simulink model "sm_stewart_platform"  (R2019b)
settings: Solver=ode45  StartTime=0.0  StopTime=450  MaxStep=0.2  RelTol=1e-3  EnableMultiTasking=on
model workspace (MAT data in the model file):
  g_density = 5
values from neighbouring files (symbols this model uses):
  B = base_points.Data(:,:,1)    [run_this_for_sim.m]
  base_radius = 0.75*100    (= 75)    [run_this_for_sim.m]
  desired_max_angle = 10    [run_this_for_sim.m]
  desired_max_x = 0.05    [run_this_for_sim.m]
  desired_max_y = desired_max_x    (= 0.05)    [run_this_for_sim.m]
  desired_max_z = 0.05    [run_this_for_sim.m]
  initial_integral_force = 200    [run_this_for_sim.m]
  leg_max = leg_min+0.3    (= 1.322)    [run_this_for_sim.m]
  leg_min = 1.022    [run_this_for_sim.m]
  leg_thickness = 75/1000    (= 0.075)    [run_this_for_sim.m]
  lower_leg_length = upper_leg_length    (= 0.511)    [run_this_for_sim.m]
  max_velocity = 0.15    [run_this_for_sim.m]
  P = platform_points.Data(:,:,1)    [run_this_for_sim.m]
  platform_radius = 0.75*base_radius    (= 56.25)    [run_this_for_sim.m]
  platform_thickness = 0.1/8    (= 0.0125)    [run_this_for_sim.m]
  trajectory_smoothing = 1/1.5    (= 0.666666666667)    [run_this_for_sim.m]
  upper_leg_length = dead_length/2    (= 0.511)    [run_this_for_sim.m]
  work_height = 1.2*100    (= 120)    [run_this_for_sim.m]
undefined symbols (not defined in the file or in its folder): nom_length, X, Z
libraries: sp_lib x18, nesl_utility x11, sm_lib x9, simulink x2
(part 10 of 10)

== system sm_stewart_platform/Subsystem/Reference Trajectory Generator7/Euler XYZ ==
  angles : Inport
  11 : Fcn  Expr=cos(u[2])*cos(u[3])
  12 : Fcn  Expr=-cos(u[2])*sin(u[3])
  13 : Fcn  Expr=sin(u[2])
  21 : Fcn  Expr=cos(u[3])*sin(u[2])*sin(u[1])+cos(u[1])*sin(u[3])
  22 : Fcn  Expr=cos(u[1])*cos(u[3]) - sin(u[1])*sin(u[2])*sin(u[3])
  23 : Fcn  Expr=-sin(u[1])*cos(u[2])
  31 : Fcn  Expr=sin(u[1])*sin(u[3]) - cos(u[1])*cos(u[3])*sin(u[2])
  32 : Fcn  Expr=cos(u[3])*sin(u[1])+cos(u[1])*sin(u[2])*sin(u[3])
  33 : Fcn  Expr=cos(u[1])*cos(u[2])
  Mux2 : Mux  Inputs=9
  Reshape 9x1->3x3 : Reshape  OutputDimensionality=Customize  OutputDimensions=[3,3]
  R : Outport  VectorParamsAs1DForOutWhenUnconnected=off
  wires:
  angles/1 -> 23/1, 33/1, 13/1, 32/1, 22/1, 12/1, 31/1, 21/1, 11/1
  33/1 -> Mux2/9
  23/1 -> Mux2/8
  13/1 -> Mux2/7
  32/1 -> Mux2/6
  22/1 -> Mux2/5
  12/1 -> Mux2/4
  31/1 -> Mux2/3
  21/1 -> Mux2/2
  11/1 -> Mux2/1
  Mux2/1 -> Reshape 9x1->3x3/1
  Reshape 9x1->3x3/1 -> R/1

== system sm_stewart_platform/Subsystem/Reference Trajectory Generator7/Euler XYZ Derivative ==
  R : Inport
  a : Inport  Port=2
  a' : Inport  Port=3
  b' : Inport  Port=4
  c' : Inport  Port=5
  Add : Sum
  Gain : Gain  Gain=-1
  Matrix Concatenate : Concatenate  NumInputs=3  Mode=Multidimensional array  ConcatenateDimension=2
  Mux5 : Mux  Inputs=3
  Prod{1..2,4..5} (4 alike) : Product  RndMeth=Zero
  Prod3 : Product  Multiplication=Matrix(*)  RndMeth=Zero
  R1 : Selector  NumberOfDimensions=2  InputPortWidth=3  IndexOptions=Select all,Index vector (dialog)  Indices=[1 3],1  OutputSizes=1,1
  R2 : Selector  NumberOfDimensions=2  InputPortWidth=3  IndexOptions=Select all,Index vector (dialog)  Indices=[1 3],2  OutputSizes=1,1
  Skew Op : Subsystem
  Vector Concatenate : Concatenate  NumInputs=3  Mode=Multidimensional array
  Zero Col : Constant  Value=[0 0 0]'
  sin cos : Trigonometry  Operator=sincos
  R' : Outport  VectorParamsAs1DForOutWhenUnconnected=off
  wires:
  a/1 -> sin cos/1
  sin cos/1 -> Prod1/2
  sin cos/2 -> Prod2/2
  b'/1 -> Prod2/1, Prod1/1
  a'/1 -> Mux5/1
  Prod2/1 -> Mux5/2
  Prod1/1 -> Mux5/3
  Mux5/1 -> Skew Op/1(v)
  Vector Concatenate/1 -> Prod4/2, Gain/1
  R2/1 -> Prod4/1
  Gain/1 -> Prod5/2
  Zero Col/1 -> Matrix Concatenate/3
  Prod5/1 -> Matrix Concatenate/2
  Prod4/1 -> Matrix Concatenate/1
  R1/1 -> Prod5/1
  Prod3/1 -> Add/1
  Matrix Concatenate/1 -> Add/2
  Add/1 -> R'/1
  R/1 -> R1/1, Prod3/2, R2/1
  Skew Op/1(v~) -> Prod3/1
  c'/1 -> Vector Concatenate/2, Vector Concatenate/1, Vector Concatenate/3

== system sm_stewart_platform/Subsystem/Reference Trajectory Generator7/Rx sinusoid ==
  t : Inport
  Add : Sum  Inputs=|++
  Add2 : Sum  Inputs=++|
  amp1 : Gain  Gain=A
  amp2 : Gain  Gain=w*A*pi/180
  deg2rad : Gain  Gain=pi/180
  freq : Gain  Gain=w
  offset : Constant  Value=k  VectorParams1D=off
  phase : Constant  Value=p  VectorParams1D=off
  sin cos : Trigonometry  Operator=sincos
  f : Outport  VectorParamsAs1DForOutWhenUnconnected=off
  f' : Outport  Port=2  VectorParamsAs1DForOutWhenUnconnected=off
  wires:
  t/1 -> freq/1
  Add/1 -> deg2rad/1
  phase/1 -> Add/2
  amp2/1 -> f'/1
  Add2/1 -> f/1
  offset/1 -> Add2/1
  sin cos/1 -> amp1/1
  sin cos/2 -> amp2/1
  amp1/1 -> Add2/2
  freq/1 -> Add/1
  deg2rad/1 -> sin cos/1

== system sm_stewart_platform/Subsystem/Reference Trajectory Generator7/Ry sinusoid ==
  t : Inport
  Add : Sum  Inputs=|++
  Add2 : Sum  Inputs=++|
  amp1 : Gain  Gain=A
  amp2 : Gain  Gain=w*A*pi/180
  deg2rad : Gain  Gain=pi/180
  freq : Gain  Gain=w
  offset : Constant  Value=k  VectorParams1D=off
  phase : Constant  Value=p  VectorParams1D=off
  sin cos : Trigonometry  Operator=sincos
  f : Outport  VectorParamsAs1DForOutWhenUnconnected=off
  f' : Outport  Port=2  VectorParamsAs1DForOutWhenUnconnected=off
  wires:
  t/1 -> freq/1
  Add/1 -> deg2rad/1
  phase/1 -> Add/2
  amp2/1 -> f'/1
  Add2/1 -> f/1
  offset/1 -> Add2/1
  sin cos/1 -> amp1/1
  sin cos/2 -> amp2/1
  amp1/1 -> Add2/2
  freq/1 -> Add/1
  deg2rad/1 -> sin cos/1

== system sm_stewart_platform/Subsystem/Reference Trajectory Generator7/Rz sinusoid ==
  t : Inport
  Add : Sum  Inputs=|++
  Add2 : Sum  Inputs=++|
  amp1 : Gain  Gain=A
  amp2 : Gain  Gain=w*A*pi/180
  deg2rad : Gain  Gain=pi/180
  freq : Gain  Gain=w
  offset : Constant  Value=k  VectorParams1D=off
  phase : Constant  Value=p  VectorParams1D=off
  sin cos : Trigonometry  Operator=sincos
  f : Outport  VectorParamsAs1DForOutWhenUnconnected=off
  f' : Outport  Port=2  VectorParamsAs1DForOutWhenUnconnected=off
  wires:
  t/1 -> freq/1
  Add/1 -> deg2rad/1
  phase/1 -> Add/2
  amp2/1 -> f'/1
  Add2/1 -> f/1
  offset/1 -> Add2/1
  sin cos/1 -> amp1/1
  sin cos/2 -> amp2/1
  amp1/1 -> Add2/2
  freq/1 -> Add/1
  deg2rad/1 -> sin cos/1

== system sm_stewart_platform/Subsystem/Reference Trajectory Generator7/dx sinusoid ==
  t : Inport
  Add : Sum  Inputs=|++
  Add2 : Sum  Inputs=++|
  amp1 : Gain  Gain=A
  amp2 : Gain  Gain=w*A*pi/180
  deg2rad : Gain  Gain=pi/180
  freq : Gain  Gain=w
  offset : Constant  Value=k  VectorParams1D=off
  phase : Constant  Value=p  VectorParams1D=off
  sin cos : Trigonometry  Operator=sincos
  f : Outport  VectorParamsAs1DForOutWhenUnconnected=off
  f' : Outport  Port=2  VectorParamsAs1DForOutWhenUnconnected=off
  wires:
  t/1 -> freq/1
  Add/1 -> deg2rad/1
  phase/1 -> Add/2
  amp2/1 -> f'/1
  Add2/1 -> f/1
  offset/1 -> Add2/1
  sin cos/1 -> amp1/1
  sin cos/2 -> amp2/1
  amp1/1 -> Add2/2
  freq/1 -> Add/1
  deg2rad/1 -> sin cos/1

== system sm_stewart_platform/Subsystem/Reference Trajectory Generator7/dy sinusoid ==
  t : Inport
  Add : Sum  Inputs=|++
  Add2 : Sum  Inputs=++|
  amp1 : Gain  Gain=A
  amp2 : Gain  Gain=w*A*pi/180
  deg2rad : Gain  Gain=pi/180
  freq : Gain  Gain=w
  offset : Constant  Value=k  VectorParams1D=off
  phase : Constant  Value=p  VectorParams1D=off
  sin cos : Trigonometry  Operator=sincos
  f : Outport  VectorParamsAs1DForOutWhenUnconnected=off
  f' : Outport  Port=2  VectorParamsAs1DForOutWhenUnconnected=off
  wires:
  t/1 -> freq/1
  Add/1 -> deg2rad/1
  phase/1 -> Add/2
  amp2/1 -> f'/1
  Add2/1 -> f/1
  offset/1 -> Add2/1
  sin cos/1 -> amp1/1
  sin cos/2 -> amp2/1
  amp1/1 -> Add2/2
  freq/1 -> Add/1
  deg2rad/1 -> sin cos/1

== system sm_stewart_platform/Subsystem/Reference Trajectory Generator7/dz sinusoid ==
  t : Inport
  Add : Sum  Inputs=|++
  Add2 : Sum  Inputs=++|
  amp1 : Gain  Gain=A
  amp2 : Gain  Gain=w*A*pi/180
  deg2rad : Gain  Gain=pi/180
  freq : Gain  Gain=w
  offset : Constant  Value=k  VectorParams1D=off
  phase : Constant  Value=p  VectorParams1D=off
  sin cos : Trigonometry  Operator=sincos
  f : Outport  VectorParamsAs1DForOutWhenUnconnected=off
  f' : Outport  Port=2  VectorParamsAs1DForOutWhenUnconnected=off
  wires:
  t/1 -> freq/1
  Add/1 -> deg2rad/1
  phase/1 -> Add/2
  amp2/1 -> f'/1
  Add2/1 -> f/1
  offset/1 -> Add2/1
  sin cos/1 -> amp1/1
  sin cos/2 -> amp2/1
  amp1/1 -> Add2/2
  freq/1 -> Add/1
  deg2rad/1 -> sin cos/1

== system sm_stewart_platform/Subsystem/Reference Trajectory Generator8/Euler XYZ ==
  angles : Inport
  11 : Fcn  Expr=cos(u[2])*cos(u[3])
  12 : Fcn  Expr=-cos(u[2])*sin(u[3])
  13 : Fcn  Expr=sin(u[2])
  21 : Fcn  Expr=cos(u[3])*sin(u[2])*sin(u[1])+cos(u[1])*sin(u[3])
  22 : Fcn  Expr=cos(u[1])*cos(u[3]) - sin(u[1])*sin(u[2])*sin(u[3])
  23 : Fcn  Expr=-sin(u[1])*cos(u[2])
  31 : Fcn  Expr=sin(u[1])*sin(u[3]) - cos(u[1])*cos(u[3])*sin(u[2])
  32 : Fcn  Expr=cos(u[3])*sin(u[1])+cos(u[1])*sin(u[2])*sin(u[3])
  33 : Fcn  Expr=cos(u[1])*cos(u[2])
  Mux2 : Mux  Inputs=9
  Reshape 9x1->3x3 : Reshape  OutputDimensionality=Customize  OutputDimensions=[3,3]
  R : Outport  VectorParamsAs1DForOutWhenUnconnected=off
  wires:
  angles/1 -> 23/1, 33/1, 13/1, 32/1, 22/1, 12/1, 31/1, 21/1, 11/1
  33/1 -> Mux2/9
  23/1 -> Mux2/8
  13/1 -> Mux2/7
  32/1 -> Mux2/6
  22/1 -> Mux2/5
  12/1 -> Mux2/4
  31/1 -> Mux2/3
  21/1 -> Mux2/2
  11/1 -> Mux2/1
  Mux2/1 -> Reshape 9x1->3x3/1
  Reshape 9x1->3x3/1 -> R/1

== system sm_stewart_platform/Subsystem/Reference Trajectory Generator8/Euler XYZ Derivative ==
  R : Inport
  a : Inport  Port=2
  a' : Inport  Port=3
  b' : Inport  Port=4
  c' : Inport  Port=5
  Add : Sum
  Gain : Gain  Gain=-1
  Matrix Concatenate : Concatenate  NumInputs=3  Mode=Multidimensional array  ConcatenateDimension=2
  Mux5 : Mux  Inputs=3
  Prod{1..2,4..5} (4 alike) : Product  RndMeth=Zero
  Prod3 : Product  Multiplication=Matrix(*)  RndMeth=Zero
  R1 : Selector  NumberOfDimensions=2  InputPortWidth=3  IndexOptions=Select all,Index vector (dialog)  Indices=[1 3],1  OutputSizes=1,1
  R2 : Selector  NumberOfDimensions=2  InputPortWidth=3  IndexOptions=Select all,Index vector (dialog)  Indices=[1 3],2  OutputSizes=1,1
  Skew Op : Subsystem
  Vector Concatenate : Concatenate  NumInputs=3  Mode=Multidimensional array
  Zero Col : Constant  Value=[0 0 0]'
  sin cos : Trigonometry  Operator=sincos
  R' : Outport  VectorParamsAs1DForOutWhenUnconnected=off
  wires:
  a/1 -> sin cos/1
  sin cos/1 -> Prod1/2
  sin cos/2 -> Prod2/2
  b'/1 -> Prod2/1, Prod1/1
  a'/1 -> Mux5/1
  Prod2/1 -> Mux5/2
  Prod1/1 -> Mux5/3
  Mux5/1 -> Skew Op/1(v)
  Vector Concatenate/1 -> Prod4/2, Gain/1
  R2/1 -> Prod4/1
  Gain/1 -> Prod5/2
  Zero Col/1 -> Matrix Concatenate/3
  Prod5/1 -> Matrix Concatenate/2
  Prod4/1 -> Matrix Concatenate/1
  R1/1 -> Prod5/1
  Prod3/1 -> Add/1
  Matrix Concatenate/1 -> Add/2
  Add/1 -> R'/1
  R/1 -> R1/1, Prod3/2, R2/1
  Skew Op/1(v~) -> Prod3/1
  c'/1 -> Vector Concatenate/2, Vector Concatenate/1, Vector Concatenate/3

== system sm_stewart_platform/Subsystem/Reference Trajectory Generator8/Rx sinusoid ==
  t : Inport
  Add : Sum  Inputs=|++
  Add2 : Sum  Inputs=++|
  amp1 : Gain  Gain=A
  amp2 : Gain  Gain=w*A*pi/180
  deg2rad : Gain  Gain=pi/180
  freq : Gain  Gain=w
  offset : Constant  Value=k  VectorParams1D=off
  phase : Constant  Value=p  VectorParams1D=off
  sin cos : Trigonometry  Operator=sincos
  f : Outport  VectorParamsAs1DForOutWhenUnconnected=off
  f' : Outport  Port=2  VectorParamsAs1DForOutWhenUnconnected=off
  wires:
  t/1 -> freq/1
  Add/1 -> deg2rad/1
  phase/1 -> Add/2
  amp2/1 -> f'/1
  Add2/1 -> f/1
  offset/1 -> Add2/1
  sin cos/1 -> amp1/1
  sin cos/2 -> amp2/1
  amp1/1 -> Add2/2
  freq/1 -> Add/1
  deg2rad/1 -> sin cos/1

== system sm_stewart_platform/Subsystem/Reference Trajectory Generator8/Ry sinusoid ==
  t : Inport
  Add : Sum  Inputs=|++
  Add2 : Sum  Inputs=++|
  amp1 : Gain  Gain=A
  amp2 : Gain  Gain=w*A*pi/180
  deg2rad : Gain  Gain=pi/180
  freq : Gain  Gain=w
  offset : Constant  Value=k  VectorParams1D=off
  phase : Constant  Value=p  VectorParams1D=off
  sin cos : Trigonometry  Operator=sincos
  f : Outport  VectorParamsAs1DForOutWhenUnconnected=off
  f' : Outport  Port=2  VectorParamsAs1DForOutWhenUnconnected=off
  wires:
  t/1 -> freq/1
  Add/1 -> deg2rad/1
  phase/1 -> Add/2
  amp2/1 -> f'/1
  Add2/1 -> f/1
  offset/1 -> Add2/1
  sin cos/1 -> amp1/1
  sin cos/2 -> amp2/1
  amp1/1 -> Add2/2
  freq/1 -> Add/1
  deg2rad/1 -> sin cos/1

== system sm_stewart_platform/Subsystem/Reference Trajectory Generator8/Rz sinusoid ==
  t : Inport
  Add : Sum  Inputs=|++
  Add2 : Sum  Inputs=++|
  amp1 : Gain  Gain=A
  amp2 : Gain  Gain=w*A*pi/180
  deg2rad : Gain  Gain=pi/180
  freq : Gain  Gain=w
  offset : Constant  Value=k  VectorParams1D=off
  phase : Constant  Value=p  VectorParams1D=off
  sin cos : Trigonometry  Operator=sincos
  f : Outport  VectorParamsAs1DForOutWhenUnconnected=off
  f' : Outport  Port=2  VectorParamsAs1DForOutWhenUnconnected=off
  wires:
  t/1 -> freq/1
  Add/1 -> deg2rad/1
  phase/1 -> Add/2
  amp2/1 -> f'/1
  Add2/1 -> f/1
  offset/1 -> Add2/1
  sin cos/1 -> amp1/1
  sin cos/2 -> amp2/1
  amp1/1 -> Add2/2
  freq/1 -> Add/1
  deg2rad/1 -> sin cos/1

== system sm_stewart_platform/Subsystem/Reference Trajectory Generator8/dx sinusoid ==
  t : Inport
  Add : Sum  Inputs=|++
  Add2 : Sum  Inputs=++|
  amp1 : Gain  Gain=A
  amp2 : Gain  Gain=w*A*pi/180
  deg2rad : Gain  Gain=pi/180
  freq : Gain  Gain=w
  offset : Constant  Value=k  VectorParams1D=off
  phase : Constant  Value=p  VectorParams1D=off
  sin cos : Trigonometry  Operator=sincos
  f : Outport  VectorParamsAs1DForOutWhenUnconnected=off
  f' : Outport  Port=2  VectorParamsAs1DForOutWhenUnconnected=off
  wires:
  t/1 -> freq/1
  Add/1 -> deg2rad/1
  phase/1 -> Add/2
  amp2/1 -> f'/1
  Add2/1 -> f/1
  offset/1 -> Add2/1
  sin cos/1 -> amp1/1
  sin cos/2 -> amp2/1
  amp1/1 -> Add2/2
  freq/1 -> Add/1
  deg2rad/1 -> sin cos/1

== system sm_stewart_platform/Subsystem/Reference Trajectory Generator8/dy sinusoid ==
  t : Inport
  Add : Sum  Inputs=|++
  Add2 : Sum  Inputs=++|
  amp1 : Gain  Gain=A
  amp2 : Gain  Gain=w*A*pi/180
  deg2rad : Gain  Gain=pi/180
  freq : Gain  Gain=w
  offset : Constant  Value=k  VectorParams1D=off
  phase : Constant  Value=p  VectorParams1D=off
  sin cos : Trigonometry  Operator=sincos
  f : Outport  VectorParamsAs1DForOutWhenUnconnected=off
  f' : Outport  Port=2  VectorParamsAs1DForOutWhenUnconnected=off
  wires:
  t/1 -> freq/1
  Add/1 -> deg2rad/1
  phase/1 -> Add/2
  amp2/1 -> f'/1
  Add2/1 -> f/1
  offset/1 -> Add2/1
  sin cos/1 -> amp1/1
  sin cos/2 -> amp2/1
  amp1/1 -> Add2/2
  freq/1 -> Add/1
  deg2rad/1 -> sin cos/1

== system sm_stewart_platform/Subsystem/Reference Trajectory Generator8/dz sinusoid ==
  t : Inport
  Add : Sum  Inputs=|++
  Add2 : Sum  Inputs=++|
  amp1 : Gain  Gain=A
  amp2 : Gain  Gain=w*A*pi/180
  deg2rad : Gain  Gain=pi/180
  freq : Gain  Gain=w
  offset : Constant  Value=k  VectorParams1D=off
  phase : Constant  Value=p  VectorParams1D=off
  sin cos : Trigonometry  Operator=sincos
  f : Outport  VectorParamsAs1DForOutWhenUnconnected=off
  f' : Outport  Port=2  VectorParamsAs1DForOutWhenUnconnected=off
  wires:
  t/1 -> freq/1
  Add/1 -> deg2rad/1
  phase/1 -> Add/2
  amp2/1 -> f'/1
  Add2/1 -> f/1
  offset/1 -> Add2/1
  sin cos/1 -> amp1/1
  sin cos/2 -> amp2/1
  amp1/1 -> Add2/2
  freq/1 -> Add/1
  deg2rad/1 -> sin cos/1

== system sm_stewart_platform/Stewart Platform System/Inverse Kinematics Module/Pos Computation/6-Way Column Splitter ==
  A : Inport
  Column 1 : Selector  NumberOfDimensions=2  InputPortWidth=3  IndexOptions=Select all,Index vector (dialog)  Indices=-1,1  OutputSizes=1
  Column 2 : Selector  NumberOfDimensions=2  InputPortWidth=3  IndexOptions=Select all,Index vector (dialog)  Indices=-1,2  OutputSizes=1
  Column 3 : Selector  NumberOfDimensions=2  InputPortWidth=3  IndexOptions=Select all,Index vector (dialog)  Indices=-1,3  OutputSizes=1
  Column 4 : Selector  NumberOfDimensions=2  InputPortWidth=3  IndexOptions=Select all,Index vector (dialog)  Indices=-1,4  OutputSizes=1
  Column 5 : Selector  NumberOfDimensions=2  InputPortWidth=3  IndexOptions=Select all,Index vector (dialog)  Indices=-1,5  OutputSizes=1
  Column 6 : Selector  NumberOfDimensions=2  InputPortWidth=3  IndexOptions=Select all,Index vector (dialog)  Indices=-1,6  OutputSizes=1
  Col1 : Outport  VectorParamsAs1DForOutWhenUnconnected=off
  Col2 : Outport  Port=2  VectorParamsAs1DForOutWhenUnconnected=off
  Col3 : Outport  Port=3  VectorParamsAs1DForOutWhenUnconnected=off
  Col4 : Outport  Port=4  VectorParamsAs1DForOutWhenUnconnected=off
  Col5 : Outport  Port=5  VectorParamsAs1DForOutWhenUnconnected=off
  Col6 : Outport  Port=6  VectorParamsAs1DForOutWhenUnconnected=off
  wires:
  A/1 -> Column 3/1, Column 2/1, Column 1/1, Column 4/1, Column 5/1, Column 6/1
  Column 1/1 -> Col1/1
  Column 2/1 -> Col2/1
  Column 3/1 -> Col3/1
  Column 4/1 -> Col4/1
  Column 5/1 -> Col5/1
  Column 6/1 -> Col6/1

== system sm_stewart_platform/Stewart Platform System/Inverse Kinematics Module/Vel Computation/6-Way Column Splitter ==
  A : Inport
  Column 1 : Selector  NumberOfDimensions=2  InputPortWidth=3  IndexOptions=Select all,Index vector (dialog)  Indices=-1,1  OutputSizes=1
  Column 2 : Selector  NumberOfDimensions=2  InputPortWidth=3  IndexOptions=Select all,Index vector (dialog)  Indices=-1,2  OutputSizes=1
  Column 3 : Selector  NumberOfDimensions=2  InputPortWidth=3  IndexOptions=Select all,Index vector (dialog)  Indices=-1,3  OutputSizes=1
  Column 4 : Selector  NumberOfDimensions=2  InputPortWidth=3  IndexOptions=Select all,Index vector (dialog)  Indices=-1,4  OutputSizes=1
  Column 5 : Selector  NumberOfDimensions=2  InputPortWidth=3  IndexOptions=Select all,Index vector (dialog)  Indices=-1,5  OutputSizes=1
  Column 6 : Selector  NumberOfDimensions=2  InputPortWidth=3  IndexOptions=Select all,Index vector (dialog)  Indices=-1,6  OutputSizes=1
  Col1 : Outport  VectorParamsAs1DForOutWhenUnconnected=off
  Col2 : Outport  Port=2  VectorParamsAs1DForOutWhenUnconnected=off
  Col3 : Outport  Port=3  VectorParamsAs1DForOutWhenUnconnected=off
  Col4 : Outport  Port=4  VectorParamsAs1DForOutWhenUnconnected=off
  Col5 : Outport  Port=5  VectorParamsAs1DForOutWhenUnconnected=off
  Col6 : Outport  Port=6  VectorParamsAs1DForOutWhenUnconnected=off
  wires:
  A/1 -> Column 3/1, Column 2/1, Column 1/1, Column 4/1, Column 5/1, Column 6/1
  Column 1/1 -> Col1/1
  Column 2/1 -> Col2/1
  Column 3/1 -> Col3/1
  Column 4/1 -> Col4/1
  Column 5/1 -> Col5/1
  Column 6/1 -> Col6/1

== system sm_stewart_platform/Stewart Platform System/Manipulator/Base/Skewed Hexagon ==
  Solid : sm_lib/Body Elements/Extruded Solid  GraphicAmbientColor=0.1 * [1 1 1]  BasedOnType=Density  CenterOfMass=[0 0 0]  CenterOfMassUnits=m  GraphicDiffuseColor=diffuse  ExtrusionCrossSection=cross_sect  ExtrusionCrossSectionUnits=cm  Density=g_density  DensityUnits=g/cm^3  DoExposeReferenceFrame=on  GraphicEmissiveColor=[0 0 0]  ExportEntireGeometry=off  ExtrusionLength=thick  ExtrusionLengthUnits=cm  ExtrusionType=General  SerializedFrames=<Frames/>  MarkerShape=Sphere  MarkerSize=1  GraphicType=FromGeometry  InertiaType=CalculateFromGeometry  Mass=1  MassUnits=kg  MomentsOfInertia=[1 1 1]  MomentsOfInertiaUnits=kg*m^2  PolygonNumSides=1  GraphicOpacity=1  PolygonOuterRadius=1  PolygonOuterRadiusUnits=m  ProductsOfInertia=[0 0 0]  ProductsOfInertiaUnits=kg*m^2  GraphicShininess=shininess  GraphicSpecularColor=specular  GraphicVisPropType=AdvancedVisualProperties
      settings: SourceProductName=Simscape Multibody
  Conn1 : PMIOPort  Side=Right
  connections:
  Conn1/RConn1 -- Solid/RConn1

== system sm_stewart_platform/Stewart Platform System/Manipulator/Platform/Skewed Hexagon ==
  Solid : sm_lib/Body Elements/Extruded Solid  GraphicAmbientColor=0.1 * [1 1 1]  BasedOnType=Density  CenterOfMass=[0 0 0]  CenterOfMassUnits=m  GraphicDiffuseColor=diffuse  ExtrusionCrossSection=cross_sect  ExtrusionCrossSectionUnits=cm  Density=g_density  DensityUnits=g/cm^3  DoExposeReferenceFrame=on  GraphicEmissiveColor=[0 0 0]  ExportEntireGeometry=off  ExtrusionLength=thick  ExtrusionLengthUnits=cm  ExtrusionType=General  SerializedFrames=<Frames/>  MarkerShape=Sphere  MarkerSize=1  GraphicType=FromGeometry  InertiaType=CalculateFromGeometry  Mass=1  MassUnits=kg  MomentsOfInertia=[1 1 1]  MomentsOfInertiaUnits=kg*m^2  PolygonNumSides=1  GraphicOpacity=1  PolygonOuterRadius=1  PolygonOuterRadiusUnits=m  ProductsOfInertia=[0 0 0]  ProductsOfInertiaUnits=kg*m^2  GraphicShininess=shininess  GraphicSpecularColor=specular  GraphicVisPropType=AdvancedVisualProperties
      settings: SourceProductName=Simscape Multibody
  Conn1 : PMIOPort  Side=Right
  connections:
  Conn1/RConn1 -- Solid/RConn1

== system sm_stewart_platform/Subsystem/Reference Trajectory Generator/Euler XYZ Derivative/Skew Op ==
  v : Inport
  Demux : Demux  Outputs=3
  Demux1 : Demux  Outputs=3
  Gain : Gain  Gain=-1
  Mux6 : Mux  Inputs=9
  Reshape 9x1->3x3 : Reshape  OutputDimensionality=Customize  OutputDimensions=[3,3]
  Zero : Constant  Value=0
  v~ : Outport  VectorParamsAs1DForOutWhenUnconnected=off
  wires:
  Mux6/1 -> Reshape 9x1->3x3/1
  v/1 -> Demux/1, Gain/1
  Gain/1 -> Demux1/1
  Reshape 9x1->3x3/1 -> v~/1
  Zero/1 -> Mux6/1, Mux6/5, Mux6/9
  Demux/3 -> Mux6/2
  Demux1/2 -> Mux6/3
  Demux1/3 -> Mux6/4
  Demux/1 -> Mux6/6
  Demux/2 -> Mux6/7
  Demux1/1 -> Mux6/8

== system sm_stewart_platform/Subsystem/Reference Trajectory Generator1/Euler XYZ Derivative/Skew Op ==
  v : Inport
  Demux : Demux  Outputs=3
  Demux1 : Demux  Outputs=3
  Gain : Gain  Gain=-1
  Mux6 : Mux  Inputs=9
  Reshape 9x1->3x3 : Reshape  OutputDimensionality=Customize  OutputDimensions=[3,3]
  Zero : Constant  Value=0
  v~ : Outport  VectorParamsAs1DForOutWhenUnconnected=off
  wires:
  Mux6/1 -> Reshape 9x1->3x3/1
  v/1 -> Demux/1, Gain/1
  Gain/1 -> Demux1/1
  Reshape 9x1->3x3/1 -> v~/1
  Zero/1 -> Mux6/1, Mux6/5, Mux6/9
  Demux/3 -> Mux6/2
  Demux1/2 -> Mux6/3
  Demux1/3 -> Mux6/4
  Demux/1 -> Mux6/6
  Demux/2 -> Mux6/7
  Demux1/1 -> Mux6/8

== system sm_stewart_platform/Subsystem/Reference Trajectory Generator2/Euler XYZ Derivative/Skew Op ==
  v : Inport
  Demux : Demux  Outputs=3
  Demux1 : Demux  Outputs=3
  Gain : Gain  Gain=-1
  Mux6 : Mux  Inputs=9
  Reshape 9x1->3x3 : Reshape  OutputDimensionality=Customize  OutputDimensions=[3,3]
  Zero : Constant  Value=0
  v~ : Outport  VectorParamsAs1DForOutWhenUnconnected=off
  wires:
  Mux6/1 -> Reshape 9x1->3x3/1
  v/1 -> Demux/1, Gain/1
  Gain/1 -> Demux1/1
  Reshape 9x1->3x3/1 -> v~/1
  Zero/1 -> Mux6/1, Mux6/5, Mux6/9
  Demux/3 -> Mux6/2
  Demux1/2 -> Mux6/3
  Demux1/3 -> Mux6/4
  Demux/1 -> Mux6/6
  Demux/2 -> Mux6/7
  Demux1/1 -> Mux6/8

== system sm_stewart_platform/Subsystem/Reference Trajectory Generator3/Euler XYZ Derivative/Skew Op ==
  v : Inport
  Demux : Demux  Outputs=3
  Demux1 : Demux  Outputs=3
  Gain : Gain  Gain=-1
  Mux6 : Mux  Inputs=9
  Reshape 9x1->3x3 : Reshape  OutputDimensionality=Customize  OutputDimensions=[3,3]
  Zero : Constant  Value=0
  v~ : Outport  VectorParamsAs1DForOutWhenUnconnected=off
  wires:
  Mux6/1 -> Reshape 9x1->3x3/1
  v/1 -> Demux/1, Gain/1
  Gain/1 -> Demux1/1
  Reshape 9x1->3x3/1 -> v~/1
  Zero/1 -> Mux6/1, Mux6/5, Mux6/9
  Demux/3 -> Mux6/2
  Demux1/2 -> Mux6/3
  Demux1/3 -> Mux6/4
  Demux/1 -> Mux6/6
  Demux/2 -> Mux6/7
  Demux1/1 -> Mux6/8

== system sm_stewart_platform/Subsystem/Reference Trajectory Generator4/Euler XYZ Derivative/Skew Op ==
  v : Inport
  Demux : Demux  Outputs=3
  Demux1 : Demux  Outputs=3
  Gain : Gain  Gain=-1
  Mux6 : Mux  Inputs=9
  Reshape 9x1->3x3 : Reshape  OutputDimensionality=Customize  OutputDimensions=[3,3]
  Zero : Constant  Value=0
  v~ : Outport  VectorParamsAs1DForOutWhenUnconnected=off
  wires:
  Mux6/1 -> Reshape 9x1->3x3/1
  v/1 -> Demux/1, Gain/1
  Gain/1 -> Demux1/1
  Reshape 9x1->3x3/1 -> v~/1
  Zero/1 -> Mux6/1, Mux6/5, Mux6/9
  Demux/3 -> Mux6/2
  Demux1/2 -> Mux6/3
  Demux1/3 -> Mux6/4
  Demux/1 -> Mux6/6
  Demux/2 -> Mux6/7
  Demux1/1 -> Mux6/8

== system sm_stewart_platform/Subsystem/Reference Trajectory Generator5/Euler XYZ Derivative/Skew Op ==
  v : Inport
  Demux : Demux  Outputs=3
  Demux1 : Demux  Outputs=3
  Gain : Gain  Gain=-1
  Mux6 : Mux  Inputs=9
  Reshape 9x1->3x3 : Reshape  OutputDimensionality=Customize  OutputDimensions=[3,3]
  Zero : Constant  Value=0
  v~ : Outport  VectorParamsAs1DForOutWhenUnconnected=off
  wires:
  Mux6/1 -> Reshape 9x1->3x3/1
  v/1 -> Demux/1, Gain/1
  Gain/1 -> Demux1/1
  Reshape 9x1->3x3/1 -> v~/1
  Zero/1 -> Mux6/1, Mux6/5, Mux6/9
  Demux/3 -> Mux6/2
  Demux1/2 -> Mux6/3
  Demux1/3 -> Mux6/4
  Demux/1 -> Mux6/6
  Demux/2 -> Mux6/7
  Demux1/1 -> Mux6/8

== system sm_stewart_platform/Subsystem/Reference Trajectory Generator7/Euler XYZ Derivative/Skew Op ==
  v : Inport
  Demux : Demux  Outputs=3
  Demux1 : Demux  Outputs=3
  Gain : Gain  Gain=-1
  Mux6 : Mux  Inputs=9
  Reshape 9x1->3x3 : Reshape  OutputDimensionality=Customize  OutputDimensions=[3,3]
  Zero : Constant  Value=0
  v~ : Outport  VectorParamsAs1DForOutWhenUnconnected=off
  wires:
  Mux6/1 -> Reshape 9x1->3x3/1
  v/1 -> Demux/1, Gain/1
  Gain/1 -> Demux1/1
  Reshape 9x1->3x3/1 -> v~/1
  Zero/1 -> Mux6/1, Mux6/5, Mux6/9
  Demux/3 -> Mux6/2
  Demux1/2 -> Mux6/3
  Demux1/3 -> Mux6/4
  Demux/1 -> Mux6/6
  Demux/2 -> Mux6/7
  Demux1/1 -> Mux6/8

== system sm_stewart_platform/Subsystem/Reference Trajectory Generator8/Euler XYZ Derivative/Skew Op ==
  v : Inport
  Demux : Demux  Outputs=3
  Demux1 : Demux  Outputs=3
  Gain : Gain  Gain=-1
  Mux6 : Mux  Inputs=9
  Reshape 9x1->3x3 : Reshape  OutputDimensionality=Customize  OutputDimensions=[3,3]
  Zero : Constant  Value=0
  v~ : Outport  VectorParamsAs1DForOutWhenUnconnected=off
  wires:
  Mux6/1 -> Reshape 9x1->3x3/1
  v/1 -> Demux/1, Gain/1
  Gain/1 -> Demux1/1
  Reshape 9x1->3x3/1 -> v~/1
  Zero/1 -> Mux6/1, Mux6/5, Mux6/9
  Demux/3 -> Mux6/2
  Demux1/2 -> Mux6/3
  Demux1/3 -> Mux6/4
  Demux/1 -> Mux6/6
  Demux/2 -> Mux6/7
  Demux1/1 -> Mux6/8

== matlab function sm_stewart_platform/Subsystem/Select scenario number/MATLAB Function ==
  data: u input; y output
function y = fcn(u)
tmp = 1;
t1 = 36;

if u >= t1
    tmp = tmp +1;
end
if u >= 2*t1
    tmp = tmp +1;
end
if u >= 3*t1
    tmp = tmp +1;
end
if u >= 4*t1
    tmp = tmp +1;
end
if u >= 5*t1
    tmp = tmp +1;
end
if u >= 6*t1
    tmp = tmp +1;
end
if u >= 7*t1
    tmp = tmp +1;
end
if u >= 8*t1
    tmp = tmp +1;
end
if u >= 9*t1
    tmp = tmp +1;
end
if u >= 10*t1
    tmp = tmp +1;
end
if u >= 11*t1
    tmp = tmp +1;
end
if u >= 12*t1
    tmp = tmp +1;
end

y = tmp;

== matlab function sm_stewart_platform/Stewart Platform System/Inertial Position Sensor/MATLAB Function ==
  data: u input; y output
function y = fcn(u)

y = quat2eul(u','XYZ');
